simulink model "test_loopback_mux_old"  (Simulink 7.0)
settings: Solver=ode45  StartTime=0.0  StopTime=4000  RelTol=1e-3
libraries: xbsIndex_r4 x329, xbsReplacements_r4 x30, xps_library x18, casper_library x9
(part 3 of 3)

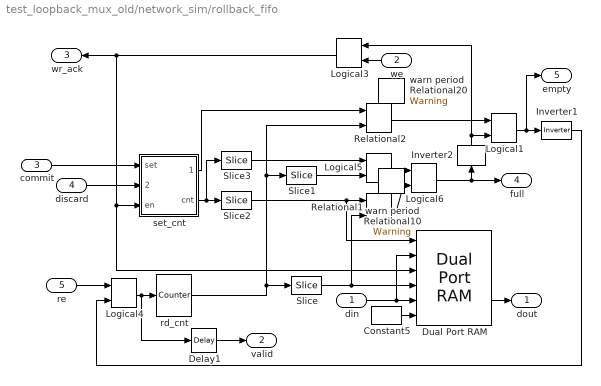
== system test_loopback_mux_old/network_sim/rollback_fifo ==
  din : Inport  OutDataType=sfix(16)  OutScaling=2^0
  we : Inport  Orientation=left  Port=2  OutDataType=sfix(16)  OutScaling=2^0
  commit : Inport  Port=3  OutDataType=sfix(16)  OutScaling=2^0
  discard : Inport  Port=4  OutDataType=sfix(16)  OutScaling=2^0
  re : Inport  Port=5  OutDataType=sfix(16)  OutScaling=2^0
  Constant5 : xbsIndex_r4/Constant  arith_type=Boolean  const=0  n_bits=1  bin_pt=0  explicit_period=on  period=1  equ=P=C  opselect=C  inp2=PCIN>>17  opr=+  inp1=P  carry=CIN  dbl_ovrd=off  block_type=constant
  Delay1 : xbsIndex_r4/Delay  en=off  latency=1  dbl_ovrd=off  reg_retiming=off  block_type=delay
      settings: xl_area=[0, 0, 0, 0, 0, 0, 0]
  Dual Port RAM : xbsIndex_r4/Dual Port RAM  depth=2^depth_bits  initVector=0  distributed_mem=Block RAM  init_a=0  init_b=0  rst_a=off  rst_b=off  en_a=off  en_b=off  latency=1  write_mode_A=Read Before Write  write_mode_B=Read Before Write  dbl_ovrd=off  optimize=Area  use_rpm=off  block_type=dpram
      settings: xl_area=[0, 0, 0, 0, 0, 0, 0]  block_version=10.1.3
  Inverter1 : xbsIndex_r4/Inverter  en=off  latency=0  dbl_ovrd=off  block_type=inv
      settings: xl_area=[0, 0, 0, 0, 0, 0, 0]
  Inverter2 : xbsIndex_r4/Inverter  Orientation=up  en=off  latency=0  dbl_ovrd=off  block_type=inv
      settings: xl_area=[0, 0, 0, 0, 0, 0, 0]
  Logical1 : xbsIndex_r4/Logical  logical_function=AND  inputs=2  en=off  latency=0  precision=Full  arith_type=Unsigned  n_bits=8  bin_pt=2  align_bp=on  dbl_ovrd=off  block_type=logical
      settings: xl_area=[0, 0, 0, 0, 0, 0, 0]
  Logical3 : xbsIndex_r4/Logical  Orientation=left  logical_function=AND  inputs=2  en=off  latency=0  precision=Full  arith_type=Unsigned  n_bits=8  bin_pt=2  align_bp=on  dbl_ovrd=off  block_type=logical
      settings: xl_area=[0, 0, 0, 0, 0, 0, 0]
  Logical4 : xbsIndex_r4/Logical  logical_function=AND  inputs=2  en=off  latency=0  precision=Full  arith_type=Unsigned  n_bits=8  bin_pt=2  align_bp=on  dbl_ovrd=off  block_type=logical
      settings: xl_area=[0, 0, 0, 0, 0, 0, 0]
  Logical5 : xbsIndex_r4/Logical  logical_function=XOR  inputs=2  en=off  latency=0  precision=Full  arith_type=Unsigned  n_bits=8  bin_pt=2  align_bp=on  dbl_ovrd=off  block_type=logical
      settings: xl_area=[0, 0, 0, 0, 0, 0, 0]
  Logical6 : xbsIndex_r4/Logical  logical_function=AND  inputs=2  en=off  latency=0  precision=Full  arith_type=Unsigned  n_bits=8  bin_pt=2  align_bp=on  dbl_ovrd=off  block_type=logical
      settings: xl_area=[0, 0, 0, 0, 0, 0, 0]
  Relational1 : xbsIndex_r4/Relational  mode=a=b  en=off  latency=0  dbl_ovrd=off  block_type=relational
      settings: xl_area=[0, 0, 0, 0, 0, 0, 0]  block_version=10.1.3
  Relational2 : xbsIndex_r4/Relational  mode=a=b  en=off  latency=0  dbl_ovrd=off  block_type=relational
      settings: xl_area=[0, 0, 0, 0, 0, 0, 0]  block_version=10.1.3
  Slice : xbsIndex_r4/Slice  nbits=1  boolean_output=off  mode=Two Bit Locations  bit1=-1  base1=MSB of Input  bit0=0  base0=LSB of Input  dbl_ovrd=off  block_type=slice
      settings: infoedit="Extracts a given range of bits from each input sample and presents it at the output.  The output type is ordinarily unsigned with binary point at zero, but can be Boolean when the slice is one bit wide.<P><P>Hardware notes: In hardware this block costs nothing."  block_version=10.1.3
  Slice1 : xbsIndex_r4/Slice  nbits=1  boolean_output=on  mode=Upper Bit Location + Width  bit1=0  base1=MSB of Input  bit0=0  base0=LSB of Input  dbl_ovrd=off  block_type=slice
      settings: infoedit="Extracts a given range of bits from each input sample and presents it at the output.  The output type is ordinarily unsigned with binary point at zero, but can be Boolean when the slice is one bit wide.<P><P>Hardware notes: In hardware this block costs nothing."  block_version=10.1.3
  Slice2 : xbsIndex_r4/Slice  nbits=1  boolean_output=off  mode=Two Bit Locations  bit1=-1  base1=MSB of Input  bit0=0  base0=LSB of Input  dbl_ovrd=off  block_type=slice
      settings: infoedit="Extracts a given range of bits from each input sample and presents it at the output.  The output type is ordinarily unsigned with binary point at zero, but can be Boolean when the slice is one bit wide.<P><P>Hardware notes: In hardware this block costs nothing."  block_version=10.1.3
  Slice3 : xbsIndex_r4/Slice  nbits=1  boolean_output=on  mode=Upper Bit Location + Width  bit1=0  base1=MSB of Input  bit0=0  base0=LSB of Input  dbl_ovrd=off  block_type=slice
      settings: infoedit="Extracts a given range of bits from each input sample and presents it at the output.  The output type is ordinarily unsigned with binary point at zero, but can be Boolean when the slice is one bit wide.<P><P>Hardware notes: In hardware this block costs nothing."  block_version=10.1.3
  rd_cnt : xbsIndex_r4/Counter  cnt_type=Free Running  cnt_to=Inf  operation=Up  start_count=0  cnt_by_val=1  arith_type=Unsigned  n_bits=depth_bits + 1  bin_pt=0  load_pin=off  rst=off  en=on  explicit_period=on  period=1  dbl_ovrd=off  use_behavioral_HDL=off  use_rpm=on  implementation=Fabric  block_type=counter
      settings: xl_area=[0, 0, 0, 0, 0, 0, 0]
  set_cnt : Subsystem
  warn period Relational10 : xbsReplacements_r4/Warning  SystemSampleTime=-1  period=1
  warn period Relational20 : xbsReplacements_r4/Warning  SystemSampleTime=-1  period=1
  dout : Outport  OutDataType=sfix(16)  OutScaling=2^0
  valid : Outport  Port=2  OutDataType=sfix(16)  OutScaling=2^0
  wr_ack : Outport  Orientation=left  Port=3  OutDataType=sfix(16)  OutScaling=2^0
  full : Outport  Port=4  OutDataType=sfix(16)  OutScaling=2^0
  empty : Outport  Port=5  OutDataType=sfix(16)  OutScaling=2^0
  wires:
  Delay1/1 -> valid/1
  Logical4/1 -> Delay1/1, rd_cnt/1
  re/1 -> Logical4/1
  Inverter1/1 -> Logical4/2
  Logical1/1 -> empty/1, Inverter1/1
  Dual Port RAM/2 -> dout/1
  Constant5/1 -> Dual Port RAM/6
  discard/1 -> set_cnt/2(undo)
  Logical3/1 -> set_cnt/3(en), Dual Port RAM/3, wr_ack/1
  we/1 -> Logical3/2
  Inverter2/1 -> Logical3/1, Logical1/2
  commit/1 -> set_cnt/1(set)
  rd_cnt/1 -> Slice/1, Slice1/1, Relational2/2
  set_cnt/1(set_cnt) -> Relational2/1
  set_cnt/2(cnt) -> Slice3/1, Slice2/1
  Slice/1 -> Dual Port RAM/4, Relational1/2
  din/1 -> Dual Port RAM/5, Dual Port RAM/2
  Slice2/1 -> Dual Port RAM/1, Relational1/1
  Slice3/1 -> Logical5/1
  Slice1/1 -> Logical5/2
  Relational1/1 -> Logical6/2
  Logical5/1 -> Logical6/1
  Logical6/1 -> full/1, Inverter2/1
  Relational2/1 -> Logical1/1

== system test_loopback_mux_old/loopback/rollback_fifo/set_cnt ==
  set : Inport  OutDataType=sfix(16)  OutScaling=2^0
  undo : Inport  Port=2  OutDataType=sfix(16)  OutScaling=2^0
  en : Inport  Port=3  OutDataType=sfix(16)  OutScaling=2^0
  Counter4 : xbsIndex_r4/Counter  cnt_type=Free Running  cnt_to=Inf  operation=Up  start_count=0  cnt_by_val=1  arith_type=Unsigned  n_bits=depth_bits + 1  bin_pt=0  load_pin=on  rst=off  en=on  explicit_period=on  period=1  dbl_ovrd=off  use_behavioral_HDL=off  use_rpm=on  implementation=Fabric  block_type=counter
      settings: xl_area=[0, 0, 0, 0, 0, 0, 0]
  Inverter : xbsIndex_r4/Inverter  en=off  latency=0  dbl_ovrd=off  block_type=inv
      settings: xl_area=[0, 0, 0, 0, 0, 0, 0]
  Inverter1 : xbsIndex_r4/Inverter  en=off  latency=0  dbl_ovrd=off  block_type=inv
      settings: xl_area=[0, 0, 0, 0, 0, 0, 0]
  Logical1 : xbsIndex_r4/Logical  logical_function=AND  inputs=3  en=off  latency=0  precision=Full  arith_type=Unsigned  n_bits=8  bin_pt=2  align_bp=on  dbl_ovrd=off  block_type=logical
      settings: xl_area=[0, 0, 0, 0, 0, 0, 0]
  Logical4 : xbsIndex_r4/Logical  logical_function=AND  inputs=3  en=off  latency=1  precision=Full  arith_type=Unsigned  n_bits=8  bin_pt=2  align_bp=on  dbl_ovrd=off  block_type=logical
      settings: xl_area=[0, 0, 0, 0, 0, 0, 0]
  Register2 : xbsIndex_r4/Register  init=0  rst=off  en=on  dbl_ovrd=off  block_type=register
      settings: xl_area=[0, 0, 0, 0, 0, 0, 0]
  set_cnt : Outport  OutDataType=sfix(16)  OutScaling=2^0
  cnt : Outport  Port=2  OutDataType=sfix(16)  OutScaling=2^0
  wires:
  Inverter1/1 -> Logical1/3
  Inverter/1 -> Logical4/3
  undo/1 -> Inverter/1, Logical1/1
  Logical1/1 -> Counter4/1
  set/1 -> Logical4/1
  Logical4/1 -> Inverter1/1, Register2/2
  Register2/1 -> set_cnt/1, Counter4/2
  en/1 -> Logical4/2, Logical1/2, Counter4/3
  Counter4/1 -> Register2/1, cnt/1

== system test_loopback_mux_old/network_sim/rollback_fifo/set_cnt ==
  set : Inport  OutDataType=sfix(16)  OutScaling=2^0
  undo : Inport  Port=2  OutDataType=sfix(16)  OutScaling=2^0
  en : Inport  Port=3  OutDataType=sfix(16)  OutScaling=2^0
  Counter4 : xbsIndex_r4/Counter  cnt_type=Free Running  cnt_to=Inf  operation=Up  start_count=0  cnt_by_val=1  arith_type=Unsigned  n_bits=depth_bits + 1  bin_pt=0  load_pin=on  rst=off  en=on  explicit_period=on  period=1  dbl_ovrd=off  use_behavioral_HDL=off  use_rpm=on  implementation=Fabric  block_type=counter
      settings: xl_area=[0, 0, 0, 0, 0, 0, 0]
  Inverter : xbsIndex_r4/Inverter  en=off  latency=0  dbl_ovrd=off  block_type=inv
      settings: xl_area=[0, 0, 0, 0, 0, 0, 0]
  Inverter1 : xbsIndex_r4/Inverter  en=off  latency=0  dbl_ovrd=off  block_type=inv
      settings: xl_area=[0, 0, 0, 0, 0, 0, 0]
  Logical1 : xbsIndex_r4/Logical  logical_function=AND  inputs=3  en=off  latency=0  precision=Full  arith_type=Unsigned  n_bits=8  bin_pt=2  align_bp=on  dbl_ovrd=off  block_type=logical
      settings: xl_area=[0, 0, 0, 0, 0, 0, 0]
  Logical4 : xbsIndex_r4/Logical  logical_function=AND  inputs=3  en=off  latency=1  precision=Full  arith_type=Unsigned  n_bits=8  bin_pt=2  align_bp=on  dbl_ovrd=off  block_type=logical
      settings: xl_area=[0, 0, 0, 0, 0, 0, 0]
  Register2 : xbsIndex_r4/Register  init=0  rst=off  en=on  dbl_ovrd=off  block_type=register
      settings: xl_area=[0, 0, 0, 0, 0, 0, 0]
  set_cnt : Outport  OutDataType=sfix(16)  OutScaling=2^0
  cnt : Outport  Port=2  OutDataType=sfix(16)  OutScaling=2^0
  wires:
  Counter4/1 -> cnt/1, Register2/1
  en/1 -> Counter4/3, Logical1/2, Logical4/2
  Register2/1 -> Counter4/2, set_cnt/1
  Logical4/1 -> Register2/2, Inverter1/1
  set/1 -> Logical4/1
  Logical1/1 -> Counter4/1
  undo/1 -> Logical1/1, Inverter/1
  Inverter/1 -> Logical4/3
  Inverter1/1 -> Logical1/3
